simulink model "TwoLinkPlanarRobotMotionControl_gen2nomfiles"  (Simulink 9.0)
settings: Solver=ode1  StartTime=0.0  StopTime=10.0  FixedStep=0.02  RelTol=1e-3  EnableMultiTasking=on
values from neighbouring files (symbols this model uses):
  m = [1 1]    [FurutaPendulum_Dynamics.m]    (also in Question_2.m = [m_1 m_2]; test_ForwardDynamics.m = [1 1 1]; test_TwoLinkPlanarRobotDynamics.m = [m1 m2]; test_TwoLinkPlanarRobotHybridControl.m = [m1 m2])
  N = 5    [createEllipsoid.m]
  s = tf('s')    [Current_loop_bode.m]    (also in Question_1.m = 15)
  X = cos(0:2*pi/n:2*pi)    [createCylinder.m]
  Y = sin(0:2*pi/n:2*pi)    [createCylinder.m]
undefined symbols (not defined in the file or in its folder): Z
libraries: sm_lib x9, nesl_utility x7
settings Model: Creator=leavesdown_admin  LastModifiedBy=leavesdown
settings DataIOCC: LimitDataPoints=on  SignalLoggingSaveFormat=ModelDataLogs
settings OptimizationCC: ExpressionDepthLimit=2147483647
settings DebuggingCC: SolverPrmCheckMsg=warning  FcnCallInpInsideContextMsg=warning  StateNameClashWarn=warning
settings GRTTargetCC: GeneratePreprocessorConditionals=Disable all
settings SimscapeCC: SimscapeNormalizeSystem=off
settings ConfigurationSet: Description=SimMechanics 2G

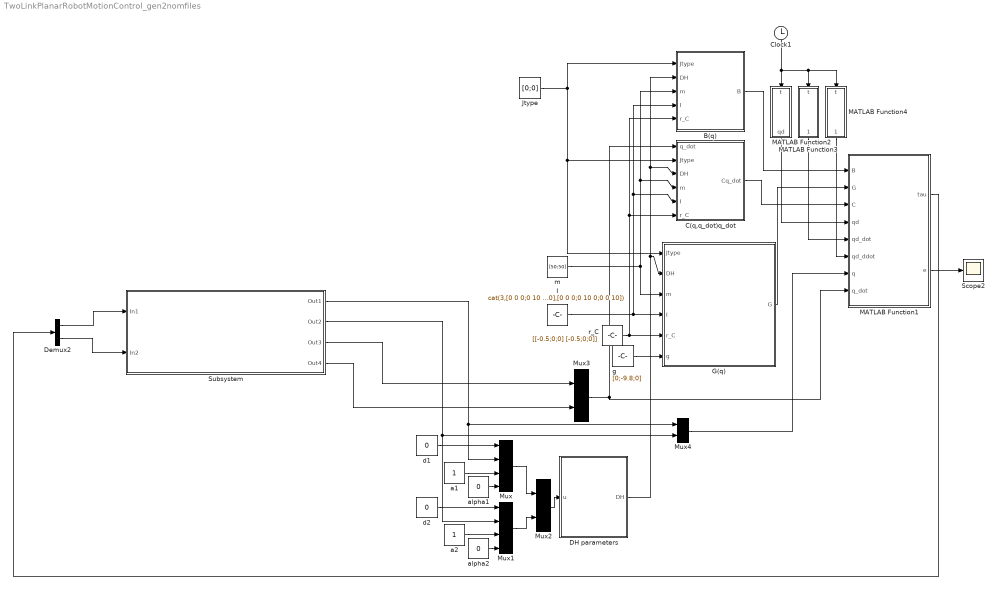
== system TwoLinkPlanarRobotMotionControl_gen2nomfiles ==
  B(q) : MATLAB Function  TreatAsAtomicUnit=on
  C(q,q_dot)q_dot : MATLAB Function  TreatAsAtomicUnit=on
  Clock1 : Clock
  DH parameters : MATLAB Function  TreatAsAtomicUnit=on
  Demux2 : Demux  Outputs=2
  G(q) : MATLAB Function  TreatAsAtomicUnit=on
  I : Constant  Value=cat(3,[0 0 0;0 10 0;0 0 10],[0 0 0;0 10 0;0 0 10])
  Jtype : Constant  Value=[0;0]
  MATLAB Function1 : MATLAB Function  TreatAsAtomicUnit=on
  MATLAB Function2 : MATLAB Function  TreatAsAtomicUnit=on
  MATLAB Function3 : MATLAB Function  TreatAsAtomicUnit=on
  MATLAB Function4 : MATLAB Function  TreatAsAtomicUnit=on
  Mux : Mux
  Mux1 : Mux
  Mux2 : Mux  Inputs=2
  Mux3 : Mux  Inputs=2
  Mux4 : Mux  Inputs=2
  Scope2 : Scope
  Subsystem : Subsystem
  a1 : Constant
  a2 : Constant
  alpha1 : Constant  Value=0
  alpha2 : Constant  Value=0
  d1 : Constant  Value=0
  d2 : Constant  Value=0
  g : Constant  Value=[0;-9.8;0]
  m : Constant  Value=[50;50]
  r_C : Constant  Value=[[-0.5;0;0] [-0.5;0;0]]
  wires:
  Demux2/1 -> Subsystem/1(In1)
  g/1 -> G(q)/6(g)
  r_C/1 -> B(q)/5(r_C), C(q,q_dot)q_dot/6(r_C), G(q)/5(r_C)
  I/1 -> B(q)/4(I), C(q,q_dot)q_dot/5(I), G(q)/4(I)
  m/1 -> B(q)/3(m), C(q,q_dot)q_dot/4(m), G(q)/3(m)
  d1/1 -> Mux/1
  a1/1 -> Mux/3
  alpha1/1 -> Mux/4
  d2/1 -> Mux1/1
  a2/1 -> Mux1/3
  alpha2/1 -> Mux1/4
  Mux/1 -> Mux2/1
  Mux1/1 -> Mux2/2
  DH parameters/1(DH) -> G(q)/2(DH), C(q,q_dot)q_dot/3(DH), B(q)/2(DH)
  Mux2/1 -> DH parameters/1(u)
  Jtype/1 -> B(q)/1(Jtype), C(q,q_dot)q_dot/2(Jtype), G(q)/1(Jtype)
  B(q)/1(B) -> MATLAB Function1/1(B)
  C(q,q_dot)q_dot/1(Cq_dot) -> MATLAB Function1/3(C)
  G(q)/1(G) -> MATLAB Function1/2(G)
  Mux3/1 -> MATLAB Function1/8(q_dot), C(q,q_dot)q_dot/1(q_dot)
  MATLAB Function2/1(qd) -> MATLAB Function1/4(qd)
  Clock1/1 -> MATLAB Function4/1(t), MATLAB Function3/1(t), MATLAB Function2/1(t)
  MATLAB Function4/1(qd_ddot) -> MATLAB Function1/6(qd_ddot)
  MATLAB Function3/1(qd_dot) -> MATLAB Function1/5(qd_dot)
  Mux4/1 -> MATLAB Function1/7(q)
  MATLAB Function1/2(e) -> Scope2/1
  MATLAB Function1/1(tau) -> Demux2/1
  Demux2/2 -> Subsystem/2(In2)
  Subsystem/1(Out1) -> Mux4/1, Mux/2
  Subsystem/2(Out2) -> Mux4/2, Mux1/2
  Subsystem/3(Out3) -> Mux3/1
  Subsystem/4(Out4) -> Mux3/2

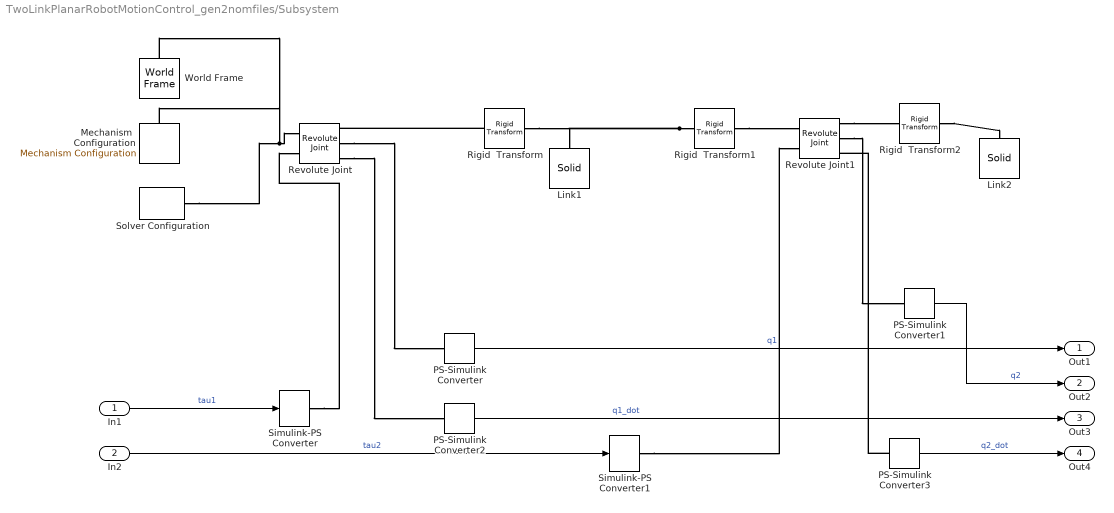
== system TwoLinkPlanarRobotMotionControl_gen2nomfiles/Subsystem ==
  In1 : Inport
  In2 : Inport  Port=2
  Link1 : sm_lib/Body Elements/Solid  InertiaType=Custom  Mass=50  MassUnits=kg  CenterOfMass=[0 0 0]  CenterOfMassUnits=m  MomentsOfInertia=[0 10 10]  MomentsOfInertiaUnits=kg*m^2  ProductsOfInertia=[0 0 0]  ProductsOfInertiaUnits=kg*m^2  DensityBased=on  Density=1000  DensityUnits=kg/(m^3)  DoExposeReferenceFrame=on  SerializedFrames=<Frames/>  GraphicType=FromGeometry  MarkerShape=Sphere  MarkerSize=10  MarkerSizeUnits=m  GraphicVisPropType=SimpleVisualProperties  GraphicDiffuseColor=[0.5 0.5 0.5]  GraphicSpecularColor=[0.5 0.5 0.5 1.0]  GraphicAmbientColor=[0.15 0.15 0.15 1.0]  GraphicEmissiveColor=[0.0 0.0 0.0 1.0]  GraphicShininess=75  GraphicOpacity=1.0  GeometryShape=Brick  RectangleSize=[1 1]  RectangleSizeUnits=m  BrickDimensions=[1 0.1 0.1]  BrickDimensionUnits=m  CylinderRadius=0.1  CylinderRadiusUnits=m  CylinderLength=1  CylinderLengthUnits=m  SphereRadius=1  SphereRadiusUnits=m  EllipsoidRadii=[1 1 1]  EllipsoidRadiiUnits=m  ExtrusionCrossSection=[1 1; -1 1; -1 -1; 1 -1]  ExtrusionCrossSectionUnits=m  ExtrusionLength=1  ExtrusionLengthUnits=m  PolygonNumSides=3  PolygonOuterRadius=1  PolygonOuterRadiusUnits=m  ExtGeomFileType=STEP  ExtGeomFileUnits=m  RevolutionCrossSection=[1 1; 1 -1; 2 -1; 2 1]  RevolutionCrossSectionUnits=m  RevolutionExtent=Full  RevolutionAngle=180  RevolutionAngleUnits=deg
  Link2 : sm_lib/Body Elements/Solid  InertiaType=Custom  Mass=50  MassUnits=kg  CenterOfMass=[0 0 0]  CenterOfMassUnits=m  MomentsOfInertia=[0 10 10]  MomentsOfInertiaUnits=kg*m^2  ProductsOfInertia=[0 0 0]  ProductsOfInertiaUnits=kg*m^2  DensityBased=on  Density=1000  DensityUnits=kg/(m^3)  DoExposeReferenceFrame=on  SerializedFrames=<Frames/>  GraphicType=FromGeometry  MarkerShape=Sphere  MarkerSize=10  MarkerSizeUnits=m  GraphicVisPropType=SimpleVisualProperties  GraphicDiffuseColor=[0.5 0.5 0.5]  GraphicSpecularColor=[0.5 0.5 0.5 1.0]  GraphicAmbientColor=[0.15 0.15 0.15 1.0]  GraphicEmissiveColor=[0.0 0.0 0.0 1.0]  GraphicShininess=75  GraphicOpacity=1.0  GeometryShape=Brick  RectangleSize=[1 1]  RectangleSizeUnits=m  BrickDimensions=[1 0.1 0.1]  BrickDimensionUnits=m  CylinderRadius=0.1  CylinderRadiusUnits=m  CylinderLength=1  CylinderLengthUnits=m  SphereRadius=1  SphereRadiusUnits=m  EllipsoidRadii=[1 1 1]  EllipsoidRadiiUnits=m  ExtrusionCrossSection=[1 1; -1 1; -1 -1; 1 -1]  ExtrusionCrossSectionUnits=m  ExtrusionLength=1  ExtrusionLengthUnits=m  PolygonNumSides=3  PolygonOuterRadius=1  PolygonOuterRadiusUnits=m  ExtGeomFileType=STEP  ExtGeomFileUnits=m  RevolutionCrossSection=[1 1; 1 -1; 2 -1; 2 1]  RevolutionCrossSectionUnits=m  RevolutionExtent=Full  RevolutionAngle=180  RevolutionAngleUnits=deg
  Mechanism  Configuration : sm_lib/Utilities/Mechanism Configuration  UniformGravity=Constant  GravityVector=[0 -9.81 0]  GravityUnits=m/s^2  LinearizationDelta=0.001
  PS-Simulink Converter{,1..3} (4 alike) : nesl_utility/PS-Simulink Converter  PhysicalDomain=network_engine_domain  SubClassName=ps_output  LeftPortType=input  RightPortType=output  PseudoPeriodic=off  Frequencies=[]  Unit=1  AffineConversion=off
  Revolute Joint : sm_lib/Joints/Revolute Joint  SenseConstraintForce=off  SenseConstraintForceX=off  SenseConstraintForceY=off  SenseConstraintForceZ=off  SenseConstraintTorque=off  SenseConstraintTorqueX=off  SenseConstraintTorqueY=off  SenseConstraintTorqueZ=off  SenseTotalForce=off  SenseTotalForceX=off  SenseTotalForceY=off  SenseTotalForceZ=off  SenseTotalTorque=off  SenseTotalTorqueX=off  SenseTotalTorqueY=off  SenseTotalTorqueZ=off  CompositeWrenchDir=FollowerOnBase  CompositeWrenchFrame=BaseFrame  EquilibriumPosition=0  EquilibriumPositionUnits=deg  SpringStiffness=0  SpringStiffnessUnits=N*m/deg  DampingCoefficient=50  DampingCoefficientUnits=N*m/(rad/s)  TorqueActuationMode=InputTorque  MotionActuationMode=ComputedMotion  SensePosition=on  SenseVelocity=on  SenseAcceleration=off  SenseTorqueForce=off  PositionTargetSpecify=on  PositionTargetPriority=High  PositionTargetValue=pi/4  PositionTargetValueUnits=rad  VelocityTargetSpecify=off  VelocityTargetPriority=High  VelocityTargetValue=0  VelocityTargetValueUnits=deg/s
  Revolute Joint1 : sm_lib/Joints/Revolute Joint  SenseConstraintForce=off  SenseConstraintForceX=off  SenseConstraintForceY=off  SenseConstraintForceZ=off  SenseConstraintTorque=off  SenseConstraintTorqueX=off  SenseConstraintTorqueY=off  SenseConstraintTorqueZ=off  SenseTotalForce=off  SenseTotalForceX=off  SenseTotalForceY=off  SenseTotalForceZ=off  SenseTotalTorque=off  SenseTotalTorqueX=off  SenseTotalTorqueY=off  SenseTotalTorqueZ=off  CompositeWrenchDir=FollowerOnBase  CompositeWrenchFrame=BaseFrame  EquilibriumPosition=0  EquilibriumPositionUnits=deg  SpringStiffness=0  SpringStiffnessUnits=N*m/deg  DampingCoefficient=50  DampingCoefficientUnits=N*m/(rad/s)  TorqueActuationMode=InputTorque  MotionActuationMode=ComputedMotion  SensePosition=on  SenseVelocity=on  SenseAcceleration=off  SenseTorqueForce=off  PositionTargetSpecify=on  PositionTargetPriority=High  PositionTargetValue=0  PositionTargetValueUnits=rad  VelocityTargetSpecify=off  VelocityTargetPriority=High  VelocityTargetValue=0  VelocityTargetValueUnits=deg/s
  Rigid  Transform : sm_lib/Frames and Transforms/Rigid Transform  TranslationMethod=Cartesian  TranslationStandardOffset=0  TranslationLengthUnit=m  TranslationStandardAxis=+Z  TranslationCartesianOffset=[0.5 0 0]  TranslationROffset=0  TranslationROffsetUnits=m  TranslationZOffset=0  TranslationZOffsetUnits=m  TranslationThetaOffset=0  TranslationThetaOffsetUnits=deg  RotationMethod=None  RotationAngleUnits=deg  RotationStandardAxis=+Z  RotationAngle=0  RotationArbitraryAxis=[0 0 1]  FollAlignAxisA=+X  BaseAlignAxisA=+Y  FollAlignAxisB=+Y  BaseAlignAxisB=+Z  RotationSequenceAxes=FollowerAxes  RotationSequence=XYX  RotationSequenceAngles=[0 0 0]  RotationSequenceAnglesUnits=deg  RotationMatrix=[1 0 0; 0 1 0; 0 0 1]
  Rigid  Transform1 : sm_lib/Frames and Transforms/Rigid Transform  TranslationMethod=Cartesian  TranslationStandardOffset=0  TranslationLengthUnit=m  TranslationStandardAxis=+Z  TranslationCartesianOffset=[0.5 0 0]  TranslationROffset=0  TranslationROffsetUnits=m  TranslationZOffset=0  TranslationZOffsetUnits=m  TranslationThetaOffset=0  TranslationThetaOffsetUnits=deg  RotationMethod=None  RotationAngleUnits=deg  RotationStandardAxis=+Z  RotationAngle=0  RotationArbitraryAxis=[0 0 1]  FollAlignAxisA=+X  BaseAlignAxisA=+Y  FollAlignAxisB=+Y  BaseAlignAxisB=+Z  RotationSequenceAxes=FollowerAxes  RotationSequence=XYX  RotationSequenceAngles=[0 0 0]  RotationSequenceAnglesUnits=deg  RotationMatrix=[1 0 0; 0 1 0; 0 0 1]
  Rigid  Transform2 : sm_lib/Frames and Transforms/Rigid Transform  TranslationMethod=Cartesian  TranslationStandardOffset=0  TranslationLengthUnit=m  TranslationStandardAxis=+Z  TranslationCartesianOffset=[0.5 0 0]  TranslationROffset=0  TranslationROffsetUnits=m  TranslationZOffset=0  TranslationZOffsetUnits=m  TranslationThetaOffset=0  TranslationThetaOffsetUnits=deg  RotationMethod=None  RotationAngleUnits=deg  RotationStandardAxis=+Z  RotationAngle=0  RotationArbitraryAxis=[0 0 1]  FollAlignAxisA=+X  BaseAlignAxisA=+Y  FollAlignAxisB=+Y  BaseAlignAxisB=+Z  RotationSequenceAxes=FollowerAxes  RotationSequence=XYX  RotationSequenceAngles=[0 0 0]  RotationSequenceAnglesUnits=deg  RotationMatrix=[1 0 0; 0 1 0; 0 0 1]
  Simulink-PS Converter : nesl_utility/Simulink-PS Converter  PhysicalDomain=network_engine_domain  SubClassName=ps_input  LeftPortType=input  RightPortType=output  PseudoPeriodic=off  Frequencies=[]  NoiseDistribution=none  NoiseParameters=[]  Unit=1  AffineConversion=off  FilteringAndDerivatives=zero  SimscapeFilterOrder=1  InputFilterTimeConstant=.001  UdotUserProvided=[]
  Simulink-PS Converter1 : nesl_utility/Simulink-PS Converter  PhysicalDomain=network_engine_domain  SubClassName=ps_input  LeftPortType=input  RightPortType=output  PseudoPeriodic=off  Frequencies=[]  NoiseDistribution=none  NoiseParameters=[]  Unit=1  AffineConversion=off  FilteringAndDerivatives=zero  SimscapeFilterOrder=1  InputFilterTimeConstant=.001  UdotUserProvided=[]
  Solver Configuration : nesl_utility/Solver Configuration  PhysicalDomain=network_engine_domain  SubClassName=solver  LeftPortType=input  RightPortType=generic  Accelerate=off  Tones=[]  Harmonics=[]  SimulateNoise=off  Profile=off  UseLocalSampling=off  EnableSwitchedLinearOptims=on  FrequencyDomain=off  UseCCode=off  RelTol=0.001  AbsTol=1e-06  MinStep=1e-09  ToWorkspace=off  RevertToSquareIcSolve=off  NumHomotopyIterations=100  PhasorMode=off  PhasorModeNumHarmonics=1  DoDC=off  ResidualTolerance=1e-9  UseLocalSolver=off  LocalSolverChoice=NE_BACKWARD_EULER_ADVANCER  LocalSolverSampleTime=.01  DoFixedCost=off  MaxNonlinIter=3  MaxModeIter=2  LinearAlgebra=Sparse  DelaysMemoryBudget=1024  AutomaticFiltering=on  FilteringTimeConstant=0.001
  World Frame : sm_lib/Frames and Transforms/World Frame
  Out1 : Outport
  Out2 : Outport  Port=2
  Out3 : Outport  Port=3
  Out4 : Outport  Port=4
  wires:
  PS-Simulink Converter1/1 -> Out2/1  "q2"
  PS-Simulink Converter/1 -> Out1/1  "q1"
  PS-Simulink Converter3/1 -> Out4/1  "q2_dot"
  In2/1 -> Simulink-PS Converter1/1  "tau2"
  PS-Simulink Converter2/1 -> Out3/1  "q1_dot"
  In1/1 -> Simulink-PS Converter/1  "tau1"
  connections:
  Rigid  Transform1/LConn1 -- Link1/RConn1 -- Rigid  Transform/RConn1
  Solver Configuration/RConn1 -- World Frame/RConn1 -- Mechanism  Configuration/RConn1 -- Revolute Joint/LConn1
  Simulink-PS Converter/RConn1 -- Revolute Joint/LConn2
  PS-Simulink Converter3/LConn1 -- Revolute Joint1/RConn3
  Rigid  Transform/LConn1 -- Revolute Joint/RConn1
  Revolute Joint/RConn2 -- PS-Simulink Converter/LConn1
  Rigid  Transform1/RConn1 -- Revolute Joint1/LConn1
  Simulink-PS Converter1/RConn1 -- Revolute Joint1/LConn2
  Rigid  Transform2/RConn1 -- Link2/RConn1
  Revolute Joint1/RConn1 -- Rigid  Transform2/LConn1
  Revolute Joint1/RConn2 -- PS-Simulink Converter1/LConn1
  Revolute Joint/RConn3 -- PS-Simulink Converter2/LConn1

== matlab function B(q) ==
  data: Jtype input double; B output double; DH input double; m input double; I input double; r_C input double
function B = fcn(Jtype,DH,m,I,r_C)
coder.extrinsic('Newton_Euler_Iteration');
n=length(m);%number of joints

B=zeros(n,n);
for i=1:n
    q_ddot_temp=[0;0];
    q_ddot_temp(i)=1;
    B(:,i) = Newton_Euler_Iteration(DH, m, I, r_C, Jtype, zeros(n,1), q_ddot_temp,zeros(3,1));
end

== matlab function C(q,q_dot)q_dot ==
  data: q_dot input double; Jtype input double; Cq_dot output double; DH input double; m input double; I input double; r_C input double
function Cq_dot = fcn(q_dot,Jtype,DH,m,I,r_C)
coder.extrinsic('Newton_Euler_Iteration');
n=length(m);%number of joints
Cq_dot=zeros(n,1);
Cq_dot=Newton_Euler_Iteration(DH, m, I, r_C, Jtype, q_dot, zeros(n,1), zeros(3,1));%compute C(q,\dot{q})\dot{q}

== matlab function G(q) ==
  data: Jtype input double; G output double; DH input double; m input double; I input double; r_C input double; g input double
function G = fcn(Jtype,DH,m,I,r_C,g)
coder.extrinsic('Newton_Euler_Iteration');
n=length(m);%number of joints
G=zeros(n,1);
G=Newton_Euler_Iteration(DH, m, I, r_C, Jtype, zeros(n,1), zeros(n,1), g);%compute C(q,\dot{q})\dot{q}

== matlab function DH parameters ==
  data: DH output double; u input double
function DH = fcn(u)
temp=reshape(u,4,length(u)/4);
DH=temp;

== matlab function MATLAB Function1 ==
  data: tau output double; B input double; G input double; C input double; qd input double; qd_dot input double; qd_ddot input double; q input double; q_dot input double; e output double
function [tau,e] = fcn(B,G,C,qd,qd_dot,qd_ddot,q,q_dot)
Kp=25.*eye(2);Kd=5.*eye(2);
kv=[50;50];
e=q-qd;e_dot=q_dot-qd_dot;
tau=-B*Kp*e-B*Kd*e_dot+G+C+kv.*q_dot+B*qd_ddot;

== matlab function MATLAB Function2 ==
  data: t input double; qd output double
function qd = fcn(t)

qd = [pi/2-pi/4*cos(2*pi/2*t);pi/4*sin(2*pi/2*t)];

== matlab function MATLAB Function3 ==
  data: t input double; qd_dot output double
function qd_dot = fcn(t)

qd_dot = [pi/4*2*pi/2*sin(2*pi/2*t);pi/4*2*pi/2*cos(2*pi/2*t)];

== matlab function MATLAB Function4 ==
  data: t input double; qd_ddot output double
function qd_ddot = fcn(t)

qd_ddot = [pi/4*((2*pi/2)^2)*cos(2*pi/2*t); -pi/4*((2*pi/2)^2)*sin(2*pi/2*t)];
